simulink model "bicopter"  (R2021b)
settings: Solver=VariableStepAuto  StartTime=0.0  StopTime=10.0  RelTol=1e-3
settings Model: Creator=KIIT  LastModifiedBy=aniruddha

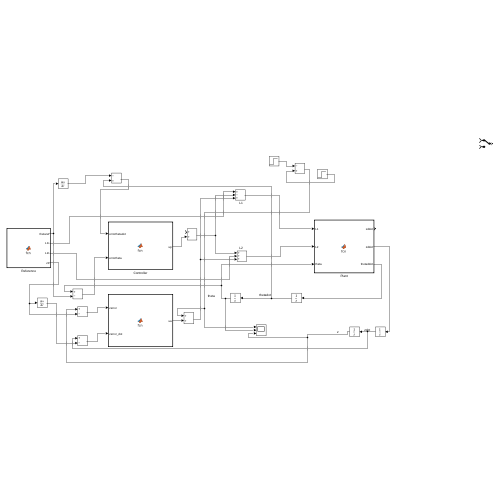
[thumbnail: Simulink's stored preview of the top-level diagram]
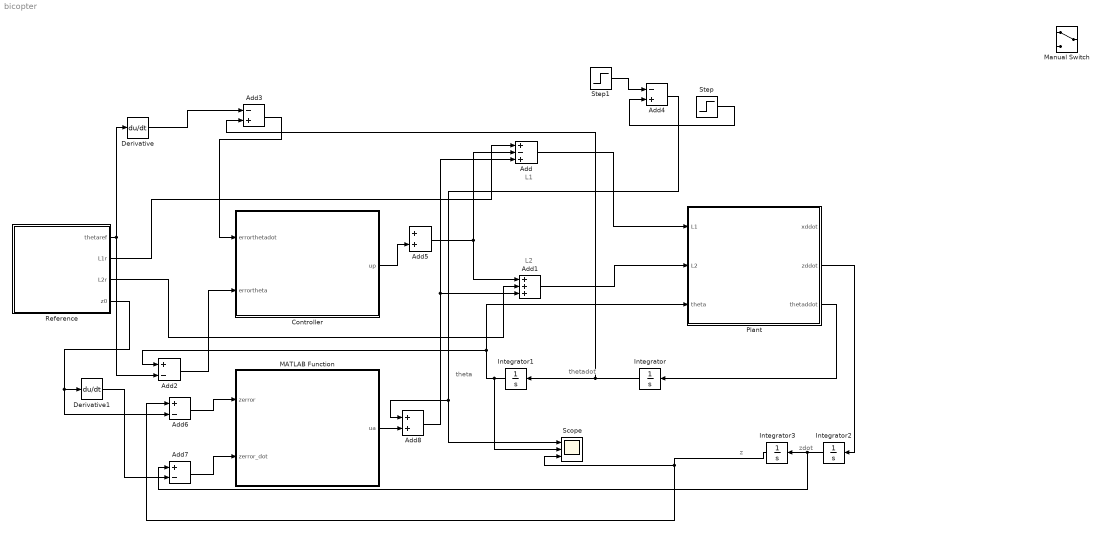
== system bicopter ==
  note: z
  note: zdot
  note: L2
  note: L1
  note: theta
  note: thetadot
  Add : Sum  Inputs=+-+
  Add1 : Sum  Inputs=+++
  Add2 : Sum  Inputs=+-
  Add3 : Sum  Inputs=-+
  Add4 : Sum  Inputs=-+
  Add5 : Sum
  Add6 : Sum  Inputs=+-
  Add7 : Sum  Inputs=+-
  Add8 : Sum
  Controller : MATLAB Function  TreatAsAtomicUnit=on
  Derivative : Derivative
  Derivative1 : Derivative
  Integrator : Integrator
  Integrator1 : Integrator  InitialCondition=pi/6.0
  Integrator2 : Integrator
  Integrator3 : Integrator
  MATLAB Function : MATLAB Function  TreatAsAtomicUnit=on
  Manual Switch : ManualSwitch
  Plant : MATLAB Function  TreatAsAtomicUnit=on
  Reference : MATLAB Function  TreatAsAtomicUnit=on
  Scope : Scope  NumInputPorts=3
  Step : Step  SampleTime=0
  Step1 : Step  Time=2  SampleTime=0
  wires:
  Controller/1(up) -> Add5/2
  Reference/2(L1r) -> Add/1
  Reference/3(L2r) -> Add1/2
  Add/1 -> Plant/1(L1)
  Add1/1 -> Plant/2(L2)
  Plant/3(thetaddot) -> Integrator/1
  Integrator/1 -> Add3/2, Integrator1/1
  Integrator1/1 -> Scope/2, Plant/3(theta), Add2/1
  Reference/1(thetaref) -> Add2/2, Derivative/1
  Derivative/1 -> Add3/1
  Add3/1 -> Controller/1(errorthetadot)
  Add2/1 -> Controller/2(errortheta)
  Step1/1 -> Add4/1
  Step/1 -> Add4/2
  Add4/1 -> Add8/1, Scope/1
  Add5/1 -> Add/2, Add1/1
  Plant/2(zddot) -> Integrator2/1
  Integrator2/1 -> Add7/1, Integrator3/1
  Reference/4(z0) -> Add6/2, Derivative1/1
  Integrator3/1 -> Scope/3, Add6/1
  Derivative1/1 -> Add7/2
  Add7/1 -> MATLAB Function/2(zerror_dot)
  Add6/1 -> MATLAB Function/1(zerror)
  MATLAB Function/1(ua) -> Add8/2
  Add8/1 -> Add/3, Add1/3

== matlab function bicopter/Plant ==
  data: L1 input; xddot output; L2 input; theta input; zddot output; thetaddot output
function [xddot, zddot, thetaddot] = fcn(L1, L2, theta)
m = 2;
Iy = 0.2;
g = 9.8;
d = 0.2;
k1 = 24;
k2 = 7;
o1 = -(1/m)*(L1+L2)*sin(theta);
o2 = (1/m)*(m*g - (L1+L2)*cos(theta));
o3 =(1/Iy)*d*(L1-L2);
xddot = o1;
zddot = o2;
thetaddot = o3;

== matlab function bicopter/Controller ==
  data: errorthetadot input; up output; errortheta input
function up  = fcn(errorthetadot, errortheta)
m = 2;
Iy = 0.2;
g = 9.8;
d = 0.2;
k1 = 24;
k2 = 7;
up = (Iy/(2*d))*((1+k1)*errortheta + k2*errorthetadot);

== matlab function bicopter/Reference ==
  data: thetaref output; L1r output; L2r output; z0 output
function [thetaref, L1r, L2r, z0] = fcn()
m = 2;
Iy = 0.2;
g = 9.8;
d = 0.2;
k1 = 24;
k2 = 7;
u = [0, m*g/2, m*g/2];
thetaref = 0;
L1r = m*g/2;
L2r = m*g/2;
z0 = 40;

== matlab function bicopter/MATLAB Function ==
  data: zerror input; ua output; zerror_dot input
function ua = fcn(zerror,zerror_dot)
m = 2;
g = 9.8;
d = 0.2;
k3 = 3;
k4 = 3;
ubar = m*((1+k3)*zerror+k4*zerror_dot);
ua = ubar/2.0;
